simulink model "FIG_2_2021_JEVG"  (R2021a)
settings: Solver=VariableStepAuto  StartTime=0.0  StopTime=10.0  RelTol=1e-3
settings Model: Creator=mluser  LastModifiedBy=user
settings DebuggingCC: UnconnectedInputMsg=none  UnconnectedOutputMsg=none  UnconnectedLineMsg=none
settings ModelReferenceCC: EnableRefExpFcnMdlSchedulingChecks=off
settings RTWCC: Description=Generic Real-Time Target  DLArmComputeVersion=20.02.1

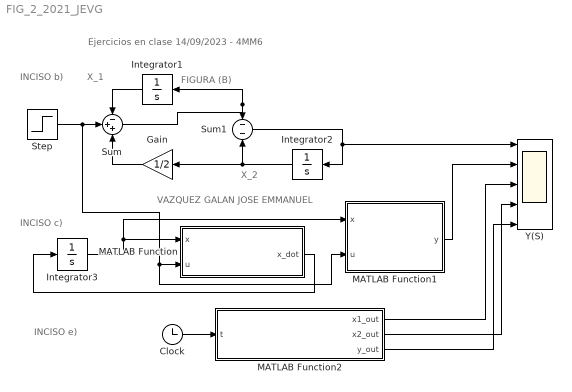
== system FIG_2_2021_JEVG ==
  note: X_2
  note: X_1
  note: VAZQUEZ GALAN JOSE EMMANUEL
  note: INCISO c)
  note: INCISO b)
  note: FIGURA (B)
  note: Ejercicios en clase 14/09/2023 - 4MM6
  note: INCISO e)
  Clock : Clock
  Gain : Gain  Gain=1/2
  Integrator1 : Integrator
  Integrator2 : Integrator
  Integrator3 : Integrator
  MATLAB Function : MATLAB Function  TreatAsAtomicUnit=on
  MATLAB Function1 : MATLAB Function  TreatAsAtomicUnit=on
  MATLAB Function2 : MATLAB Function  TreatAsAtomicUnit=on
  Step : Step  SampleTime=0
  Sum : Sum  Inputs=-++
  Sum1 : Sum  Inputs=--
  "Y(S) " : Scope  NumInputPorts=5
  wires:
  Integrator1/1 -> Sum/1
  Gain/1 -> Sum/3
  Sum/1 -> Integrator1/1, Sum1/1
  Integrator2/1 -> Sum1/2, Gain/1
  Sum1/1 -> Integrator2/1, "Y(S) "/1
  Integrator3/1 -> MATLAB Function/1(x), MATLAB Function1/1(x)
  Step/1 -> MATLAB Function1/2(u), MATLAB Function/2(u), Sum/2
  MATLAB Function1/1(y) -> "Y(S) "/2
  MATLAB Function/1(x_dot) -> Integrator3/1
  Clock/1 -> MATLAB Function2/1(t)
  MATLAB Function2/1(x1_out) -> "Y(S) "/3
  MATLAB Function2/2(x2_out) -> "Y(S) "/4
  MATLAB Function2/3(y_out) -> "Y(S) "/5

== matlab function FIG_2_2021_JEVG/MATLAB Function ==
  data: x input size=[2, 1]; u input size=[1, 1]; x_dot output size=[2, 1]
function x_dot = stateSpaceSystem(x, u)
    % Matrices A y B para el sistema dado
    A = [-1, 0.5; 1, -1.5];
    B = [1; -1];

    % Sistema en espacio de estado
    x_dot = A*x + B*u;
end

== matlab function FIG_2_2021_JEVG/MATLAB Function2 ==
  data: x1_out output; x2_out output; t input; y_out output
function [x1_out, x2_out, y_out] = stateResponse(t)
    if t < 1
        x1_out = 0;
        x2_out = 0;
        y_out = 0;
    else
        u = -1; % Valor del escalón después de t=1
        x1_out = x1_func_new(t-1) + u;
        x2_out = x2_func_new(t-1) + u;
        y_out = y_func_new(t-1) + u;
    end
end

== matlab function FIG_2_2021_JEVG/MATLAB Function1 ==
  data: x input; y output; u input
function y = outputFunction(x, u)
    % Matriz C y contribución directa D
    C = [1, -1.5];
    D = -1;

    % Cálculo de la salida
    y = C*x + D*u;
end
